simulink model "3.2"  (R2018a)
settings: Solver=ode4  StartTime=0.0  StopTime=30  FixedStep=0.001  RelTol=1e-3
undefined symbols (not defined in the file): K_alpha2az, kaz, kq, M_alpha, M_dlte, M_q, Z_alpha, Z_dlte
settings Model: Creator=80741  LastModifiedBy=80741
settings DataIOCC: LimitDataPoints=on  SaveFormat=Array  SignalLoggingSaveFormat=ModelDataLogs
settings OptimizationCC: InitFltsAndDblsToZero=on  LifeSpan=inf
settings DebuggingCC: SaveWithParameterizedLinksMsg=none  UnderspecifiedInitializationDetection=Classic  MergeDetectMultiDrivingBlocksExec=none  SignalResolutionControl=TryResolveAllWithWarning  SolverPrmCheckMsg=warning  MultiTaskDSMMsg=warning  MultiTaskCondExecSysMsg=none  FcnCallInpInsideContextMsg=warning  SFUnexpectedBacktrackingDiag=warning  SFNoUnconditionalDefaultTransitionDiag=warning  SFExecutionAtInitializationDiag=none
settings HardwareCC: ProdBitPerPointer=32  ProdBitPerSizeT=32  ProdBitPerPtrDiffT=32  ProdLargestAtomicFloat=None  ProdIntDivRoundTo=Undefined  ProdEndianess=Unspecified  ProdWordSize=32  ProdHWDeviceType=32-bit Generic
settings ModelReferenceCC: PropagateSignalLabelsOutOfModel=off
settings CodeAppCC: StateflowObjectComments=on
settings GRTTargetCC: TargetFcnLib=ansi_tfl_tmw.mat  TargetLangStandard=C89/C90 (ANSI)  CombineOutputUpdateFcns=off  GRTInterface=on
settings ConfigComp: CovMetricSettings=dw  CovHtmlReporting=on  CovSaveCumulativeToWorkspaceVar=on  CovSaveSingleToWorkspaceVar=on  CovExternalEMLEnable=off

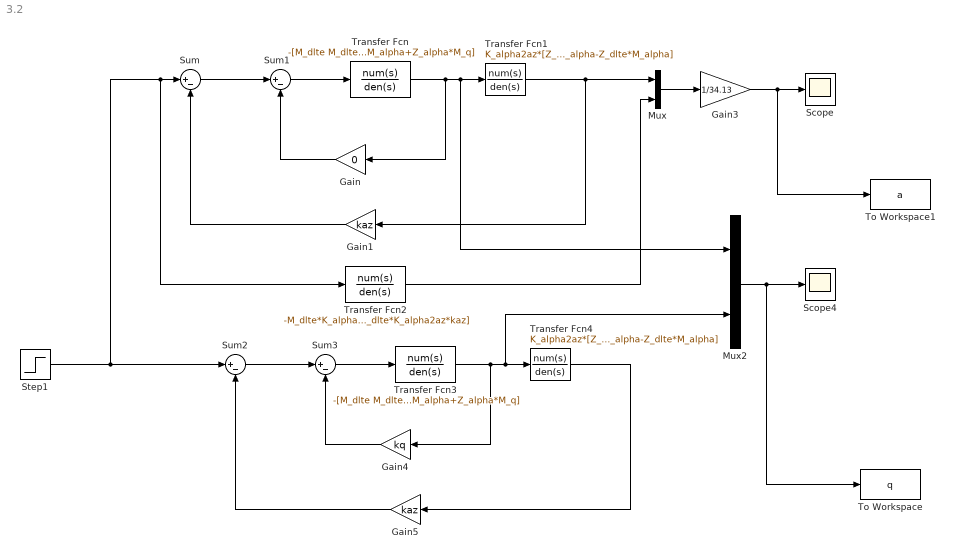
== system 3.2 ==
  Gain : Gain  Gain=0
  Gain1 : Gain  Gain=kaz
  Gain3 : Gain  Gain=1/34.13
  Gain4 : Gain  Gain=kq
  Gain5 : Gain  Gain=kaz
  Mux : Mux  Inputs=2
  Mux2 : Mux  Inputs=2
  Scope : Scope
  Scope4 : Scope
  Step1 : Step  Time=0  SampleTime=0
  Sum{,1..3} (4 alike) : Sum  Inputs=|+-
  To Workspace : ToWorkspace  VariableName=q  SaveFormat=Timeseries  SampleTime=-1
  To Workspace1 : ToWorkspace  VariableName=a  SaveFormat=Timeseries  SampleTime=-1
  Transfer Fcn : TransferFcn  Numerator=-[M_dlte M_dlte*Z_alpha-Z_dlte*M_alpha]  Denominator=[1 Z_alpha+M_q M_alpha+Z_alpha*M_q]
  Transfer Fcn1 : TransferFcn  Numerator=K_alpha2az*[Z_dlte M_dlte+Z_dlte*M_q]  Denominator=[M_dlte M_dlte*Z_alpha-Z_dlte*M_alpha]
  Transfer Fcn2 : TransferFcn  Numerator=-M_dlte*K_alpha2az  Denominator=[1 Z_alpha+M_q-M_dlte*kq M_alpha+Z_alpha*M_q-M_dlte*Z_alpha*kq-M_dlte*K_alpha2az*kaz]
  Transfer Fcn3 : TransferFcn  Numerator=-[M_dlte M_dlte*Z_alpha-Z_dlte*M_alpha]  Denominator=[1 Z_alpha+M_q M_alpha+Z_alpha*M_q]
  Transfer Fcn4 : TransferFcn  Numerator=K_alpha2az*[Z_dlte M_dlte+Z_dlte*M_q]  Denominator=[M_dlte M_dlte*Z_alpha-Z_dlte*M_alpha]
  wires:
  Step1/1 -> Sum/1, Transfer Fcn2/1, Sum2/1
  Sum/1 -> Sum1/1
  Sum1/1 -> Transfer Fcn/1
  Transfer Fcn/1 -> Gain/1, Mux2/1, Transfer Fcn1/1
  Gain/1 -> Sum1/2
  Transfer Fcn1/1 -> Gain1/1, Mux/1
  Gain1/1 -> Sum/2
  Transfer Fcn2/1 -> Mux/2
  Mux/1 -> Gain3/1
  Gain3/1 -> To Workspace1/1, Scope/1
  Gain5/1 -> Sum2/2
  Gain4/1 -> Sum3/2
  Sum2/1 -> Sum3/1
  Transfer Fcn3/1 -> Gain4/1, Mux2/2, Transfer Fcn4/1
  Sum3/1 -> Transfer Fcn3/1
  Transfer Fcn4/1 -> Gain5/1
  Mux2/1 -> To Workspace/1, Scope4/1
